simulink model "MPC_scheme_StateRegulation"  (R2025b)
settings: Solver=VariableStepAuto  StartTime=0.0  StopTime=t_sim  RelTol=1e-3
undefined symbols (not defined in the file): A, B, C, md, Ts, x0
settings Model: Creator=nicol  LastModifiedBy=nicol

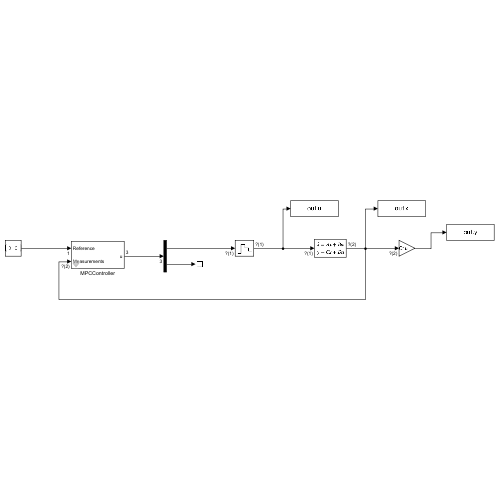
[thumbnail: Simulink's stored preview of the top-level diagram]
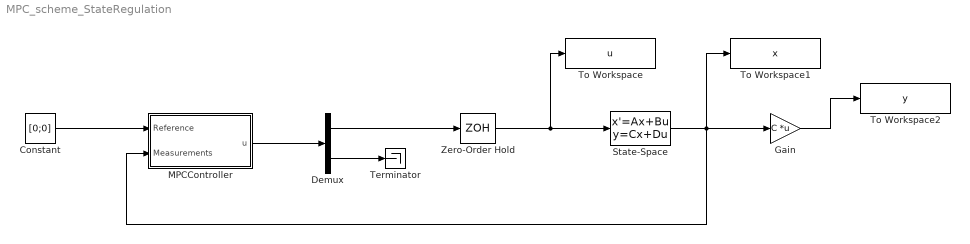
== system MPC_scheme_StateRegulation ==
  Constant : Constant  Value=[0;0]
  Demux : Demux  Outputs=2
  Gain : Gain  Gain=C  Multiplication=Matrix(K*u)
  MPCController : Subsystem  mask{md=md}
      mask prompts: md "MPCData"
  State-Space : StateSpace  A=A  B=B  C=eye(2)  D=[0;0]  InitialCondition=x0
  Terminator : Terminator
  To Workspace : ToWorkspace  VariableName=u  SaveFormat=Structure With Time  SampleTime=-1
  To Workspace1 : ToWorkspace  VariableName=x  SaveFormat=Structure With Time  SampleTime=-1
  To Workspace2 : ToWorkspace  VariableName=y  SaveFormat=Structure With Time  SampleTime=-1
  Zero-Order Hold : ZeroOrderHold  SampleTime=Ts
  wires:
  Demux/1 -> Zero-Order Hold/1
  Zero-Order Hold/1 -> To Workspace/1, State-Space/1
  Constant/1 -> MPCController/1(Reference)
  State-Space/1 -> MPCController/2(Measurements), Gain/1, To Workspace1/1
  Gain/1 -> To Workspace2/1
  MPCController/1(u) -> Demux/1
  Demux/2 -> Terminator/1

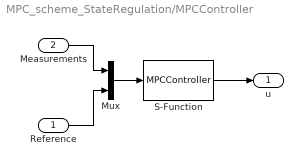
== system MPC_scheme_StateRegulation/MPCController ==
  Reference : Inport
  Measurements : Inport  Port=2
  Mux : Mux  Inputs=2
  S-Function : S-Function  FunctionName=MPCController  Parameters=md  SFunctionDeploymentMode=off  EnableBusSupport=off
  u : Outport
  wires:
  Mux/1 -> S-Function/1
  Measurements/1 -> Mux/1
  Reference/1 -> Mux/2
  S-Function/1 -> u/1
